simulink model "P5p3c"  (R2017b)
settings: Solver=ode45  StartTime=0.0  StopTime=5000  RelTol=1e-3  EnableMultiTasking=on
values from neighbouring files (symbols this model uses):
  K = 0.16    [P5p3b.m]    (also in P5p3b_init.m; P5p3c.m; P5p3d.m; P5p3d_init.m)
  K_pd = 10^((K_pd_desibel))    [P5p3b.m]    (also in P5p3b_init.m; P5p3c.m; P5p3d.m; P5p3d_init.m)
  psi_ref = 30    [P5p3b.m]    (also in P5p3b_init.m; P5p3c.m; P5p3d.m; P5p3d_init.m)
  T = 70.55    [P5p3b.m]    (also in P5p3b_init.m; P5p3c.m; P5p3d.m; P5p3d_init.m)
  T_f = 0.119*T    (= 8.39545)    [P5p3b.m]    (also in P5p3b_init.m; P5p3c.m; P5p3d.m; P5p3d_init.m)
libraries: simulink x2
settings Model: Creator=markh  LastModifiedBy=Sjurinho
settings DataIOCC: LimitDataPoints=on  SaveFormat=Array  SignalLoggingSaveFormat=ModelDataLogs  SignalLoggingName=sigsOut
settings OptimizationCC: InitFltsAndDblsToZero=on  LifeSpan=inf
settings DebuggingCC: SaveWithParameterizedLinksMsg=none  UnderspecifiedInitializationDetection=Classic  MergeDetectMultiDrivingBlocksExec=none  SignalResolutionControl=TryResolveAllWithWarning  MultiTaskDSMMsg=warning  MultiTaskCondExecSysMsg=none  FcnCallInpInsideContextMsg=warning  StateNameClashWarn=warning  StrictBusMsg=None  SFUnexpectedBacktrackingDiag=warning  SFNoUnconditionalDefaultTransitionDiag=warning  SFExecutionAtInitializationDiag=none
settings HardwareCC: ProdBitPerPointer=32  ProdBitPerSizeT=32  ProdBitPerPtrDiffT=32  ProdLargestAtomicFloat=None  ProdIntDivRoundTo=Undefined  ProdEndianess=Unspecified  ProdWordSize=32  ProdHWDeviceType=32-bit Generic  TargetUnknown=on
settings ModelReferenceCC: PropagateSignalLabelsOutOfModel=off
settings RTWCC: Description=Generic Real-Time Target
settings CodeAppCC: StateflowObjectComments=on
settings GRTTargetCC: TargetFcnLib=ansi_tfl_tmw.mat  TargetLangStandard=C89/C90 (ANSI)  GeneratePreprocessorConditionals=Disable all  CombineOutputUpdateFcns=off  GRTInterface=on
settings ConfigComp: CovMetricSettings=dw  CovHtmlReporting=on  CovSaveCumulativeToWorkspaceVar=on  CovSaveSingleToWorkspaceVar=on  CovExternalEMLEnable=off

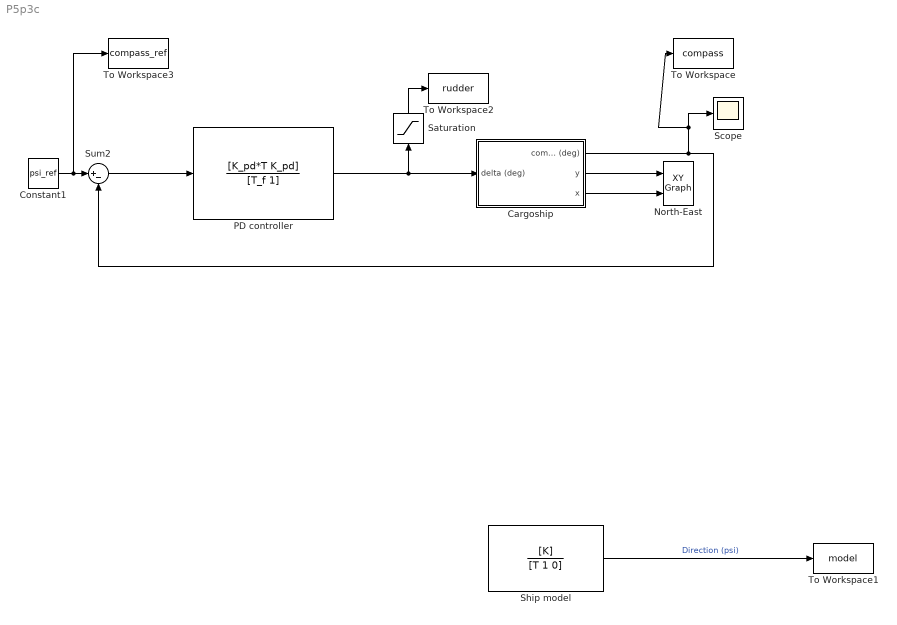
== system P5p3c ==
  Cargoship : Subsystem  mask(Simple shipmodel for a cargo ship){noise=on, current=on, logic=off}
      mask prompts: noise "measurement noise"; logic "waves"
      mask help:
      | Measurement noise:
      | 	checked = noise on
      | 	unchecked = noise off
      |
      | Current:
      | 	checked = current on
      | 	unchecked = current off
      |
      | Waves:
      | 	checked = waves on
      | 	unchecked = waves off
      |
      | Author: Jørgen Spjøtvold, 9/10-2003
      | TTK 4115 Linear system theory.
      | Modified by Jostein Bakkeheim 26/10-2006
  Constant1 : Constant  Value=psi_ref
  North-East : simulink/Sinks/XY Graph  xmin=-5000  xmax=7500  ymin=-5000  ymax=5000  st=-1
  PD controller : TransferFcn  Numerator=[K_pd*T K_pd]  Denominator=[T_f 1]
  Saturation : Saturate  UpperLimit=45  LowerLimit=-45
  Scope : Scope
  Ship model : TransferFcn  Numerator=[K]  Denominator=[T 1 0]
  Sum2 : Sum  Inputs=|+-
  To Workspace : ToWorkspace  VariableName=compass  SaveFormat=Structure With Time  SampleTime=-1
      settings: MaxDataPoints=9999999
  To Workspace1 : ToWorkspace  VariableName=model  SaveFormat=Structure With Time  SampleTime=-1
      settings: MaxDataPoints=9999999
  To Workspace2 : ToWorkspace  VariableName=rudder  SaveFormat=Structure With Time  SampleTime=-1
      settings: MaxDataPoints=9999999
  To Workspace3 : ToWorkspace  VariableName=compass_ref  SaveFormat=Structure With Time  SampleTime=-1
      settings: MaxDataPoints=9999999
  wires:
  Cargoship/3(x) -> North-East/2
  Cargoship/2(y) -> North-East/1
  Cargoship/1(compass (deg)) -> Sum2/2, Scope/1, To Workspace/1
  Ship model/1 -> To Workspace1/1  "Direction (psi)"
  Constant1/1 -> To Workspace3/1, Sum2/1
  Sum2/1 -> PD controller/1
  PD controller/1 -> Saturation/1, Cargoship/1(delta (deg))
  Saturation/1 -> To Workspace2/1

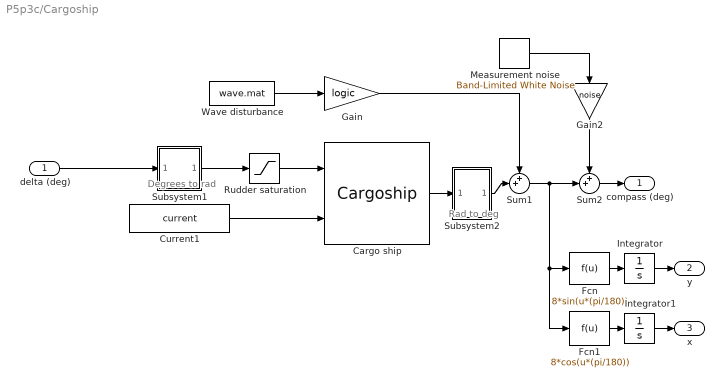
== system P5p3c/Cargoship ==
  note: Degrees to rad
  note: Rad to deg
  delta (deg) : Inport
  Cargo ship : S-Function  FunctionName=Cargoship  SFunctionDeploymentMode=off  EnableBusSupport=off  mask(Cargo ship){}
      mask help:
      | S-function which simulates a cargo ship.
      |
      | Author: Jørgen Spjøtvold
      | 20.10-2003
      | Modified by Jostein Bakkeheim 27.10.2006
  Current1 : Constant  Value=current
  Fcn : Fcn  Expr=8*sin(u*(pi/180))
  Fcn1 : Fcn  Expr=8*cos(u*(pi/180))
  Gain : Gain  Gain=logic  SaturateOnIntegerOverflow=on  OutDataTypeStr=Inherit: Same as input  ParamDataTypeStr=Inherit: Same as input
  Gain2 : Gain  Gain=noise  SaturateOnIntegerOverflow=on  OutDataTypeStr=Inherit: Same as input  ParamDataTypeStr=Inherit: Same as input
  Integrator : Integrator
  Integrator1 : Integrator
  Measurement noise : simulink/Sources/Band-Limited White Noise  Cov=[0.001]  Ts=.5  seed=[23341]
  Rudder saturation : Saturate  UpperLimit=45*(pi/180)  LowerLimit=-45*(pi/180)
  Subsystem1 : Subsystem  mask(degrees to radians){}
      mask help: Converts degrees to radians
      mask Display: fprintf('D2R');
  Subsystem2 : Subsystem  mask(radians to degrees){}
      mask help: Converts radians to degrees
      mask Display: fprintf('R2D');
  Sum1 : Sum  Inputs=++|  SaturateOnIntegerOverflow=on
  Sum2 : Sum  Inputs=++|  SaturateOnIntegerOverflow=on
  Wave disturbance : FromFile  FileName=wave.mat  SampleTime=0
  compass (deg) : Outport
  y : Outport  Port=2
  x : Outport  Port=3
  wires:
  delta (deg)/1 -> Subsystem1/1(In1)
  Fcn/1 -> Integrator/1
  Integrator/1 -> y/1
  Fcn1/1 -> Integrator1/1
  Integrator1/1 -> x/1
  Wave disturbance/1 -> Gain/1
  Subsystem2/1(Out1) -> Sum1/2
  Gain/1 -> Sum1/1
  Sum1/1 -> Fcn/1, Fcn1/1, Sum2/2
  Cargo ship/1 -> Subsystem2/1(In1)
  Subsystem1/1(Out1) -> Rudder saturation/1
  Rudder saturation/1 -> Cargo ship/1
  Sum2/1 -> compass (deg)/1
  Measurement noise/1 -> Gain2/1
  Gain2/1 -> Sum2/1
  Current1/1 -> Cargo ship/2

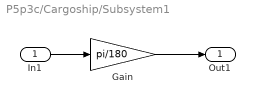
== system P5p3c/Cargoship/Subsystem1 ==
  In1 : Inport
  Gain : Gain  Gain=pi/180  SaturateOnIntegerOverflow=on  OutDataTypeStr=Inherit: Same as input  ParamDataTypeStr=Inherit: Same as input
  Out1 : Outport
  wires:
  Gain/1 -> Out1/1
  In1/1 -> Gain/1

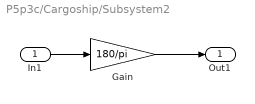
== system P5p3c/Cargoship/Subsystem2 ==
  In1 : Inport
  Gain : Gain  Gain=180/pi  SaturateOnIntegerOverflow=on  OutDataTypeStr=Inherit: Same as input  ParamDataTypeStr=Inherit: Same as input
  Out1 : Outport
  wires:
  Gain/1 -> Out1/1
  In1/1 -> Gain/1
